simulink model "Synchronous_Machine_model_Simulation"  (R2024b)
settings: Solver=ode23t  StartTime=0.0  StopTime=20  RelTol=1e-6
values from neighbouring files (symbols this model uses):
  f = 60    [Parameter synchronous machine submission.m]
  i_f = Vfd/Rpf    [Parameter synchronous machine submission.m]
  ids = 0    [Parameter synchronous machine submission.m]
  iqs = sqrt(7.9674e+03)    [Parameter synchronous machine submission.m]
  J = 35.1e6    (= 35100000)    [Parameter synchronous machine submission.m]
  JL = Jmat*L    [Parameter synchronous machine submission.m]
  L = [Lq 0 0 Lmq Lmq 0 0 ... (first row only)    [Parameter synchronous machine submission.m]
  Linv = inv(L)    [Parameter synchronous machine submission.m]
  P = 64    [Parameter synchronous machine submission.m]
  R = [Rs 0 0 0 0 0 0 ... (first row only)    [Parameter synchronous machine submission.m]
  theta_e0 = theta_r0*P/2    (= 0)    [Parameter synchronous machine submission.m]
  theta_r0 = 0    [Parameter synchronous machine submission.m]
  Vabc_s = 20e3*sqrt(2)/sqrt(3)    [Parameter synchronous machine submission.m]
  Vfd = Epf*Rpf/(Lmd*web)    [Parameter synchronous machine submission.m]
  wb = 112.5*2*pi/60    (= 11.780972451)    [Parameter synchronous machine submission.m]
settings Model: Creator=QUDUS  LastModifiedBy=krishanchoudhary
settings RTWCC: GPUComputeCapability=3.5

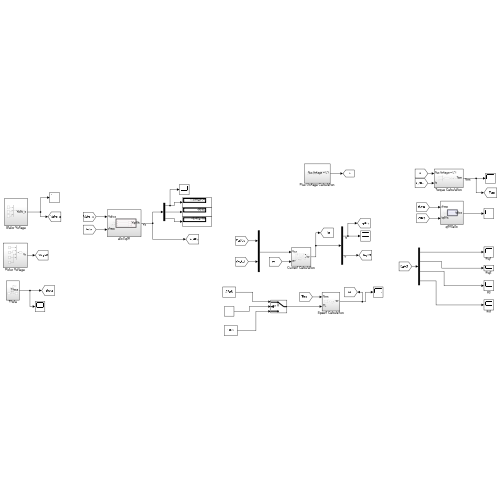
[thumbnail: Simulink's stored preview of the top-level diagram]
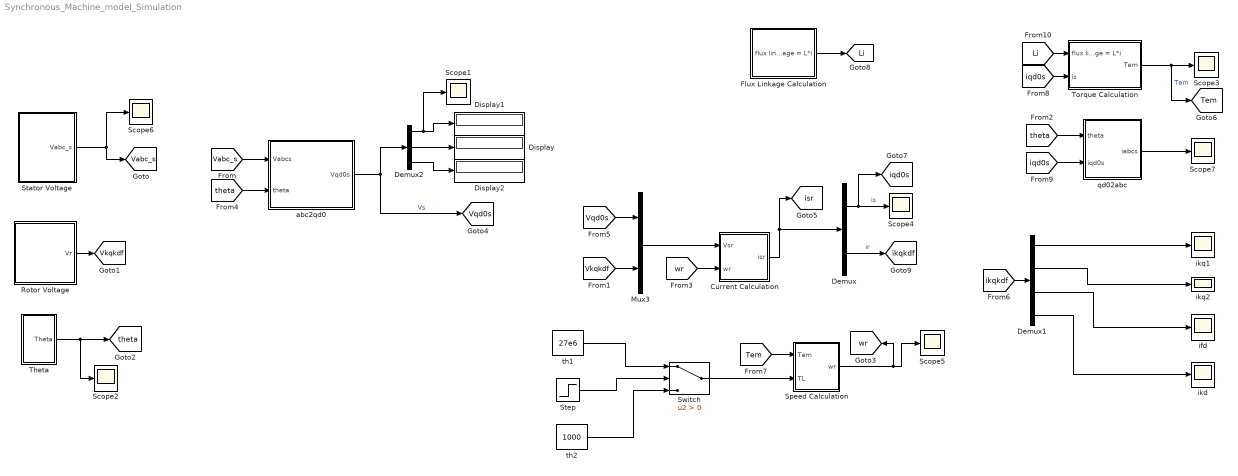
== system Synchronous_Machine_model_Simulation ==
  Current Calculation : Subsystem
  Demux : Demux  Outputs=[3 4]
  Demux1 : Demux
  Demux2 : Demux  Outputs=3
  Display : Display
  Display1 : Display
  Display2 : Display
  Flux Linkage Calculation : Subsystem
  Mux3 : Mux  Inputs=[3 4]
  Rotor Voltage : Subsystem
  Scope{1..7} (7 alike) : Scope
  Speed Calculation : Subsystem
  Stator Voltage : Subsystem
  Step : Step  Time=4  SampleTime=0
  Switch : Switch  Criteria=u2 > Threshold  SaturateOnIntegerOverflow=off  InputSameDT=off
  Theta : Subsystem
  Torque Calculation : Subsystem
  abc2qd0 : Subsystem
  ifd : Scope
  ikd : Scope
  ikq1 : Scope
  ikq2 : Scope
  qd02abc : Subsystem
  th1 : Constant  Value=27e6
  th2 : Constant  Value=1000
  tag scope: Li=global, Tem=global, Vabc_s=global, Vkqkdf=global, Vqd0s=global, ikqkdf=global, iqd0s=global, isr=global, theta=global, wr=global
  wires:
  Demux2/3 -> Display2/1
  Demux1/1 -> ikq1/1
  Demux1/4 -> ikd/1
  Torque Calculation/1(Tem) -> [Tem], Scope3/1  "Tem"
  abc2qd0/1(Vqd0s) -> [Vqd0s], Demux2/1  "Vs"
  Demux2/1 -> Scope1/1, Display1/1
  Demux2/2 -> Display/1
  Current Calculation/1(isr) -> Demux/1, [isr]
  Demux/1 -> [iqd0s], Scope4/1  "is"
  Mux3/1 -> Current Calculation/1(Vsr)
  Speed Calculation/1(wr) -> Scope5/1, [wr]
  qd02abc/1(iabcs) -> Scope7/1
  [Vabc_s] -> abc2qd0/1(Vabcs)
  [Vkqkdf] -> Mux3/2
  [theta] -> qd02abc/1(theta)
  Stator Voltage/1(Vabc_s) -> Scope6/1, [Vabc_s]
  Rotor Voltage/1(Vr) -> [Vkqkdf]
  [wr] -> Current Calculation/2(wr)
  [Vqd0s] -> Mux3/1
  Theta/1(Theta) -> Scope2/1, [theta]
  [theta] -> abc2qd0/2("theta ")
  [Tem] -> Speed Calculation/1(Tem)
  [iqd0s] -> Torque Calculation/2(is)
  [iqd0s] -> qd02abc/2(iqd0s)
  [Li] -> Torque Calculation/1(flux linkage = L*i)
  Demux1/3 -> ifd/1
  Flux Linkage Calculation/1(flux linkage = L*i) -> [Li]
  Demux/2 -> [ikqkdf]  "ir"
  [ikqkdf] -> Demux1/1
  Step/1 -> Switch/2
  th1/1 -> Switch/1
  th2/1 -> Switch/3
  Switch/1 -> Speed Calculation/2(TL)
  Demux1/2 -> ikq2/1

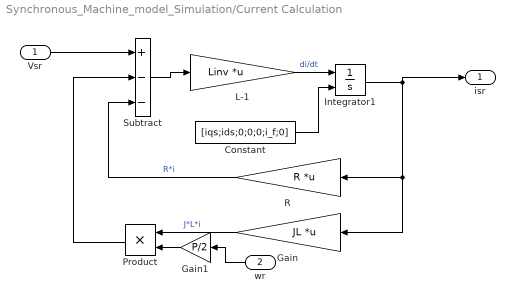
== system Synchronous_Machine_model_Simulation/Current Calculation ==
  Vsr : Inport
  wr : Inport  Port=2
  Constant : Constant  Value=[iqs;ids;0;0;0;i_f;0]
  Gain : Gain  Gain=JL  Multiplication=Matrix(K*u) (u vector)
  Gain1 : Gain  Gain=P/2
  Integrator1 : Integrator  InitialConditionSource=external  InitialCondition=[iqs;ids;0;0;0;i_f;0]
  L-1 : Gain  Gain=Linv  Multiplication=Matrix(K*u) (u vector)
  Product : Product
  R : Gain  Gain=R  Multiplication=Matrix(K*u) (u vector)
  Subtract : Sum  Inputs=+--
  isr : Outport
  wires:
  Product/1 -> Subtract/2
  Gain/1 -> Product/1  "J*L*i"
  Subtract/1 -> L-1/1
  R/1 -> Subtract/3  "R*i"
  Vsr/1 -> Subtract/1
  Gain1/1 -> Product/2
  wr/1 -> Gain1/1
  L-1/1 -> Integrator1/1  "di/dt"
  Integrator1/1 -> isr/1, Gain/1, R/1
  Constant/1 -> Integrator1/2

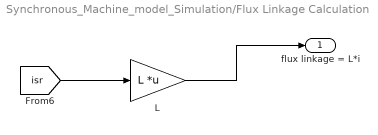
== system Synchronous_Machine_model_Simulation/Flux Linkage Calculation ==
  L : Gain  Gain=L  Multiplication=Matrix(K*u) (u vector)
  flux linkage = L*i : Outport
  wires:
  [isr] -> L/1
  L/1 -> flux linkage = L*i/1

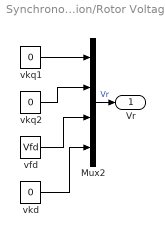
== system Synchronous_Machine_model_Simulation/Rotor Voltage ==
  Mux2 : Mux
  vfd : Constant  Value=Vfd
  vkd : Constant  Value=0
  vkq1 : Constant  Value=0
  vkq2 : Constant  Value=0
  Vr : Outport
  wires:
  vkq2/1 -> Mux2/2
  vfd/1 -> Mux2/3
  vkd/1 -> Mux2/4
  vkq1/1 -> Mux2/1
  Mux2/1 -> Vr/1  "Vr"

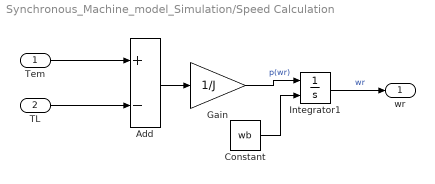
== system Synchronous_Machine_model_Simulation/Speed Calculation ==
  Tem : Inport
  TL : Inport  Port=2
  Add : Sum  Inputs=+-
  Constant : Constant  Value=wb
  Gain : Gain  Gain=1/J
  Integrator1 : Integrator  InitialConditionSource=external  InitialCondition=wb
  wr : Outport
  wires:
  Add/1 -> Gain/1
  TL/1 -> Add/2
  Gain/1 -> Integrator1/1  "p(wr)"
  Tem/1 -> Add/1
  Integrator1/1 -> wr/1  "wr"
  Constant/1 -> Integrator1/2

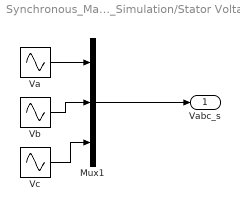
== system Synchronous_Machine_model_Simulation/Stator Voltage ==
  Mux1 : Mux  Inputs=3
  Va : Sin  Amplitude=Vabc_s  Frequency=f*2*pi  Phase=theta_e0+pi/2  SampleTime=0
  "Vb " : Sin  Amplitude=Vabc_s  Frequency=f*2*pi  Phase=theta_e0-2*pi/3+pi/2  SampleTime=0
  Vc : Sin  Amplitude=Vabc_s  Frequency=f*2*pi  Phase=theta_e0+2*pi/3+pi/2  SampleTime=0
  Vabc_s : Outport
  wires:
  Mux1/1 -> Vabc_s/1
  Vc/1 -> Mux1/3
  Va/1 -> Mux1/1
  "Vb "/1 -> Mux1/2

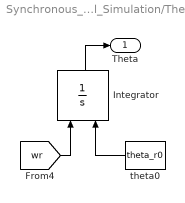
== system Synchronous_Machine_model_Simulation/Theta ==
  Integrator : Integrator  InitialConditionSource=external
  theta0 : Constant  Value=theta_r0
  Theta : Outport
  wires:
  theta0/1 -> Integrator/2
  Integrator/1 -> Theta/1
  [wr] -> Integrator/1

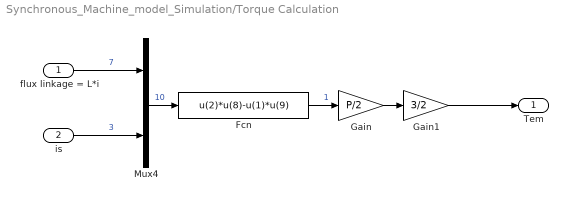
== system Synchronous_Machine_model_Simulation/Torque Calculation ==
  flux linkage = L*i : Inport
  is : Inport  Port=2
  Fcn : Fcn  Expr=u(2)*u(8)-u(1)*u(9)
  Gain : Gain  Gain=P/2
  Gain1 : Gain  Gain=3/2
  Mux4 : Mux  Inputs=[7 3]
  Tem : Outport
  wires:
  Gain1/1 -> Tem/1
  Gain/1 -> Gain1/1
  Mux4/1 -> Fcn/1  "10"
  flux linkage = L*i/1 -> Mux4/1  "7"
  Fcn/1 -> Gain/1  "1"
  is/1 -> Mux4/2  "3"

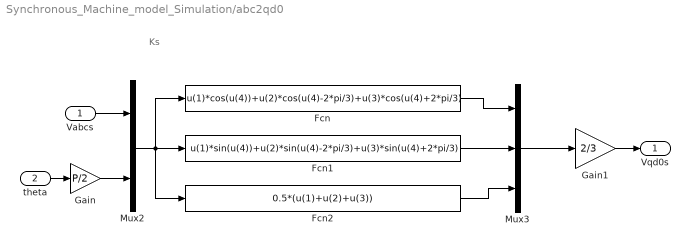
== system Synchronous_Machine_model_Simulation/abc2qd0 ==
  note: Ks
  Vabcs : Inport
  "theta " : Inport  Port=2
  Fcn : Fcn  Expr=u(1)*cos(u(4))+u(2)*cos(u(4)-2*pi/3)+u(3)*cos(u(4)+2*pi/3)
  Fcn1 : Fcn  Expr=u(1)*sin(u(4))+u(2)*sin(u(4)-2*pi/3)+u(3)*sin(u(4)+2*pi/3)
  Fcn2 : Fcn  Expr=0.5*(u(1)+u(2)+u(3))
  Gain : Gain  Gain=P/2
  Gain1 : Gain  Gain=2/3
  Mux2 : Mux  Inputs=[3 1]
  Mux3 : Mux  Inputs=3
  Vqd0s : Outport
  wires:
  Fcn/1 -> Mux3/1
  Fcn1/1 -> Mux3/2
  Mux2/1 -> Fcn2/1, Fcn1/1, Fcn/1
  Fcn2/1 -> Mux3/3
  Mux3/1 -> Gain1/1
  Gain1/1 -> Vqd0s/1
  "theta "/1 -> Gain/1
  Gain/1 -> Mux2/2
  Vabcs/1 -> Mux2/1

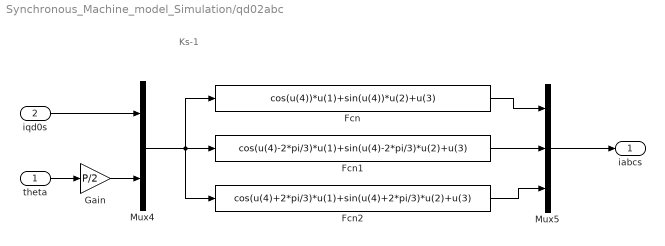
== system Synchronous_Machine_model_Simulation/qd02abc ==
  note: Ks-1
  theta : Inport
  iqd0s : Inport  Port=2
  Fcn : Fcn  Expr=cos(u(4))*u(1)+sin(u(4))*u(2)+u(3)
  Fcn1 : Fcn  Expr=cos(u(4)-2*pi/3)*u(1)+sin(u(4)-2*pi/3)*u(2)+u(3)
  Fcn2 : Fcn  Expr=cos(u(4)+2*pi/3)*u(1)+sin(u(4)+2*pi/3)*u(2)+u(3)
  Gain : Gain  Gain=P/2
  Mux4 : Mux  Inputs=[3 1]
  Mux5 : Mux  Inputs=3
  iabcs : Outport
  wires:
  iqd0s/1 -> Mux4/1
  Fcn/1 -> Mux5/1
  Mux4/1 -> Fcn2/1, Fcn1/1, Fcn/1
  Mux5/1 -> iabcs/1
  Fcn1/1 -> Mux5/2
  Fcn2/1 -> Mux5/3
  theta/1 -> Gain/1
  Gain/1 -> Mux4/2
